simulink model "q2_f"  (R2016a)
settings: Solver=VariableStepAuto  StartTime=0.0  StopTime=20  RelTol=1e-3
settings Model: Creator=pc  LastModifiedBy=pc

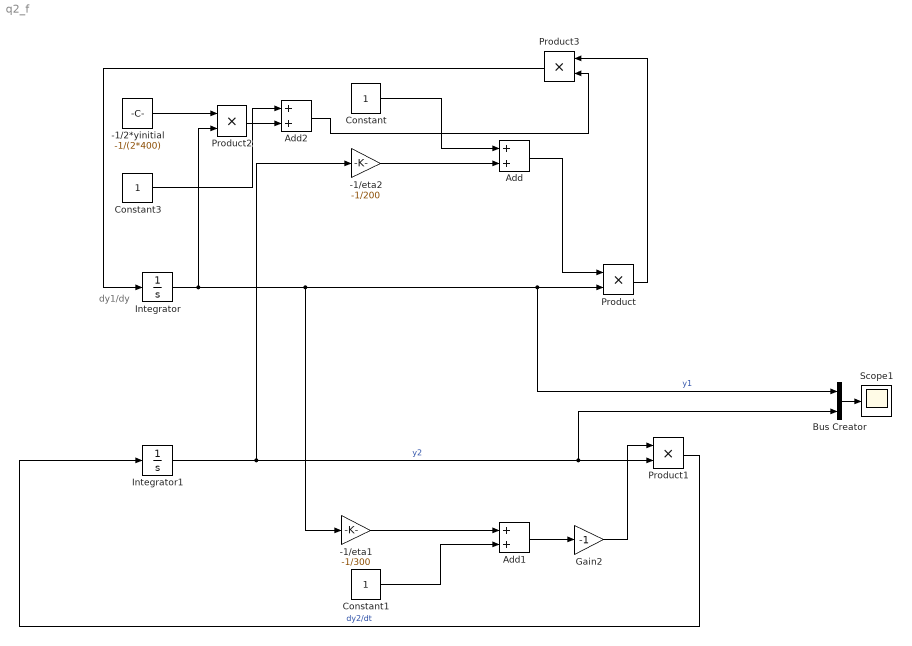
== system q2_f ==
  note: dy1/dy
  -1/2*yinitial : Constant  Value=-1/(2*400)
  -1/eta1 : Gain  Gain=-1/300
  -1/eta2 : Gain  Gain=-1/200
  Add : Sum
  Add1 : Sum
  Add2 : Sum
  Bus Creator : BusCreator  Inputs=2
  Constant : Constant
  Constant1 : Constant
  Constant3 : Constant
  Gain2 : Gain  Gain=-1
  Integrator : Integrator  InitialCondition=400
  Integrator1 : Integrator  InitialCondition=100
  Product{,1..3} (4 alike) : Product
  Scope1 : Scope
  wires:
  Integrator/1 -> Product2/2, -1/eta1/1, Bus Creator/1, Product/2  "y1"
  Integrator1/1 -> -1/eta2/1, Bus Creator/2, Product1/2  "y2"
  -1/eta2/1 -> Add/2
  Constant/1 -> Add/1
  Add/1 -> Product/1
  -1/eta1/1 -> Add1/1
  Constant1/1 -> Add1/2
  Add1/1 -> Gain2/1
  Gain2/1 -> Product1/1
  Product1/1 -> Integrator1/1  "dy2/dt"
  Bus Creator/1 -> Scope1/1
  -1/2*yinitial/1 -> Product2/1
  Product2/1 -> Add2/2
  Constant3/1 -> Add2/1
  Product/1 -> Product3/1
  Add2/1 -> Product3/2
  Product3/1 -> Integrator/1
